simulink model "Exp13_CCCV"  (R2022b)
settings: Solver=VariableStepAuto  StartTime=0.0  StopTime=3600  RelTol=1e-3
undefined symbols (not defined in the file or in its folder): Ion, Lithium
libraries: spsBatteryLib x3, BatteryCurrentManagement x2, spsControlledCurrentSourceLib x2, spsDiodeLib x2, spsIdealSwitchLib x2, spsSeriesRLCBranchLib x2, spsGroundLib x1, BatteryBalancing x1, sps_lib x1
settings Model: Creator=SASTRA  LastModifiedBy=SASTRA
settings SolverCC: MaxConsecutiveMinStep=100

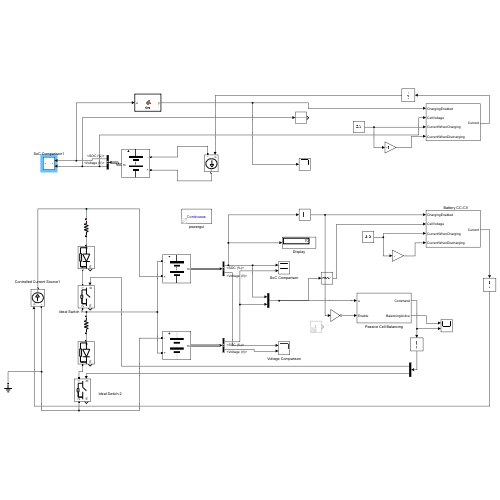
[thumbnail: Simulink's stored preview of the top-level diagram]
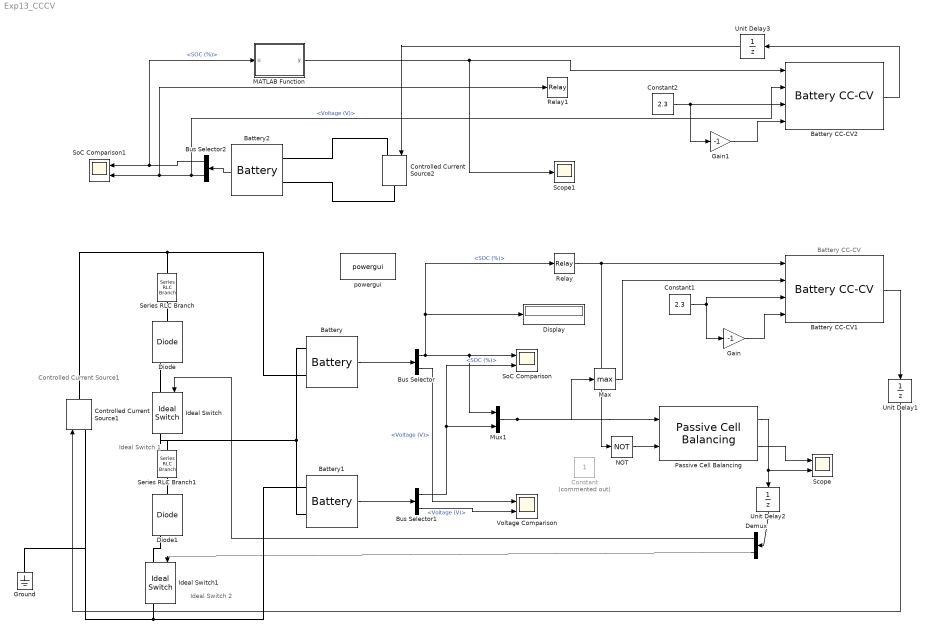
== system Exp13_CCCV ==
  note: Ideal Switch 1
  note: Ideal Switch 2
  note: Controlled Current Source1
  note: Battery CC-CV
  Battery : spsBatteryLib/Battery  BatType=Lithium-Ion  ShowTempParam=off  ThermalPreset="3.3V  2.3Ah  (LiFePO4)"  ShowAgeParam=off  NomV=3.1  NomQ=2.3  SOC=70  Batt_Tr=1  PresetModel=off  MaxQ=2.3  MinV=3.75  FullV=3.748  Dis_rate=2.3  R=0.014  Normal_OP=2.25  expZone="[3.4788       0.113]"  current=[6.5 13 32.5]  Units=Time  Tci=20  NomT=25  T2=0  MaxQ2=2.208  FullV2=3.45  Normal_OP2=2.85  expZone2="[3.22       0.015]"  Rca=0.6  ti=1000  Dp=0  Neq0=0  Tsim=1e6  Ta1=25  Qeol=5.4*0.9  Reol=0.013333*1.2  Char_age=[2.3478, 3]  Dis_age=[2.3478, 10]  N1=1500  N2=10500  N3=1000  N4=1400  Ta2=45  N5=950
  Battery CC-CV1 : BatteryCurrentManagement/Battery CC-CV  MaxCellVoltage=4.5  Kp=100  Ki=10  Kaw=1  Ts=1
      settings: LibrarySourceBlock=batt_sl_lib/Current Management/Battery CC-CV
  Battery CC-CV2 : BatteryCurrentManagement/Battery CC-CV  MaxCellVoltage=4.5  Kp=100  Ki=10  Kaw=1  Ts=1
      settings: LibrarySourceBlock=batt_sl_lib/Current Management/Battery CC-CV
  Battery1 : spsBatteryLib/Battery  BatType=Lithium-Ion  ShowTempParam=off  ThermalPreset="3.3V  2.3Ah  (LiFePO4)"  ShowAgeParam=off  NomV=3.1  NomQ=2.3  SOC=50  Batt_Tr=1  PresetModel=off  MaxQ=2.3  MinV=2.475  FullV=3.748  Dis_rate=2.3  R=0.014  Normal_OP=2.25  expZone="[3.4788       0.113]"  current=[6.5 13 32.5]  Units=Time  Tci=20  NomT=25  T2=0  MaxQ2=2.208  FullV2=3.45  Normal_OP2=2.85  expZone2="[3.22       0.015]"  Rca=0.6  ti=1000  Dp=0  Neq0=0  Tsim=1e6  Ta1=25  Qeol=5.4*0.9  Reol=0.013333*1.2  Char_age=[2.3478, 3]  Dis_age=[2.3478, 10]  N1=1500  N2=10500  N3=1000  N4=1400  Ta2=45  N5=950
  Battery2 : spsBatteryLib/Battery  BatType=Lithium-Ion  ShowTempParam=off  ThermalPreset="3.3V  2.3Ah  (LiFePO4)"  ShowAgeParam=off  NomV=3.1  NomQ=2.3  SOC=70  Batt_Tr=1  PresetModel=off  MaxQ=2.3  MinV=3.75  FullV=3.748  Dis_rate=2.3  R=0.014  Normal_OP=2.25  expZone="[3.4788       0.113]"  current=[6.5 13 32.5]  Units=Time  Tci=20  NomT=25  T2=0  MaxQ2=2.208  FullV2=3.45  Normal_OP2=2.85  expZone2="[3.22       0.015]"  Rca=0.6  ti=1000  Dp=0  Neq0=0  Tsim=1e6  Ta1=25  Qeol=5.4*0.9  Reol=0.013333*1.2  Char_age=[2.3478, 3]  Dis_age=[2.3478, 10]  N1=1500  N2=10500  N3=1000  N4=1400  Ta2=45  N5=950
  Bus Selector : BusSelector  OutputSignals=SOC (%),Voltage (V)
  Bus Selector1 : BusSelector  OutputSignals=SOC (%),Voltage (V)
  Bus Selector2 : BusSelector  OutputSignals=SOC (%),Voltage (V)
  Constant : Constant  Commented=on
  Constant1 : Constant  Value=2.3
  Constant2 : Constant  Value=2.3
  Controlled Current Source1 : spsControlledCurrentSourceLib/Controlled Current Source  Initialize=on  Source_Type=DC  Amplitude=0  Phase=0  Frequency=0  Measurements=Current
  Controlled Current Source2 : spsControlledCurrentSourceLib/Controlled Current Source  Initialize=on  Source_Type=DC  Amplitude=0  Phase=0  Frequency=0  Measurements=Current
  Demux : Demux  Outputs=2
  Diode : spsDiodeLib/Diode  Ron=0.001  Lon=0  Vf=0.8  IC=0  UseSnubber=0  Rs=500  Cs=250e-9  Measurements=on
  Diode1 : spsDiodeLib/Diode  Ron=0.001  Lon=0  Vf=0.8  IC=0  UseSnubber=0  Rs=500  Cs=250e-9  Measurements=on
  Display : Display
  Gain : Gain  Gain=-1
  Gain1 : Gain  Gain=-1
  Ground : spsGroundLib/Ground  LConnTagsString=a
  Ideal Switch : spsIdealSwitchLib/Ideal Switch  Ron=0.001  Lon=0  IC=0  Rs=1e5  Cs=inf  Measurements=on
  Ideal Switch1 : spsIdealSwitchLib/Ideal Switch  Ron=0.001  Lon=0  IC=0  Rs=1e5  Cs=inf  Measurements=on
  MATLAB Function : MATLAB Function  TreatAsAtomicUnit=on
  Max : MinMax  Function=max
  Mux1 : Mux  Inputs=2
  NOT : Logic  Operator=NOT  IconShape=distinctive  AllPortsSameDT=off  OutDataTypeStr=boolean
  Passive Cell Balancing : BatteryBalancing/Passive Cell Balancing  Threshold=0.2  Td_on=1  Td_off=1  Ts=1
      settings: LibrarySourceBlock=batt_sl_lib/Cell Balancing/Passive Cell Balancing
  Relay : Relay  OnSwitchValue=90  OffSwitchValue=30  OnOutputValue=0  OffOutputValue=1
  Relay1 : Relay  OnSwitchValue=3.3  OffSwitchValue=3.2
  Scope : Scope  NumInputPorts=2
  Scope1 : Scope
  Series RLC Branch : spsSeriesRLCBranchLib/Series RLC Branch  LConnTagsString=__new0  RConnTagsString=__new0  BranchType=R  Resistance=10  Inductance=1e-3  SetiL0=off  InitialCurrent=0  Capacitance=1e-6  Setx0=off  InitialVoltage=0  Measurements=None
  Series RLC Branch1 : spsSeriesRLCBranchLib/Series RLC Branch  LConnTagsString=__new0  RConnTagsString=__new0  BranchType=R  Resistance=10  Inductance=1e-3  SetiL0=off  InitialCurrent=0  Capacitance=1e-6  Setx0=off  InitialVoltage=0  Measurements=None
  SoC Comparison : Scope  NumInputPorts=2
  SoC Comparison1 : Scope  NumInputPorts=2
  Unit Delay1 : UnitDelay  SampleTime=-1  HasFrameUpgradeWarning=on
  Unit Delay2 : UnitDelay  SampleTime=-1  HasFrameUpgradeWarning=on
  Unit Delay3 : UnitDelay  SampleTime=-1  HasFrameUpgradeWarning=on
  Voltage Comparison : Scope  NumInputPorts=2
  powergui : sps_lib/powergui  Priority=1  SimulationMode=Continuous  SampleTime=50e-6  frequency=60  Iterations=50  frequencyindice=0  Pbase=100e6  ErrMax=1e-4  UnitsV=kV  UnitsW=MW  buscounter=0  FunctionMessages=off  echomessages=off  EnableUseOfTLC=off  CurrentSourceSwitches=off  DisableSnubberDevices=off  DisableRonSwitches=off  DisableVfSwitches=off  DisplayEquations=off  AutomaticDiscreteSolvers=off  SolverType=Tustin/Backward Euler (TBE)  Interpol=off  ExternalGateDelay=off  methode=off  Ts=100  x0status=blocks  SPID=on  SwTol=0  HookPort=off  NonlinearTolerance=1e-4  nMaxIteration=100  ContinueOnMaxIteration=off  RestoreLinks=warning  ResistiveCurrentMeasurement=off  Frange=[0:2:500]  Ylog=off  Xlog=on  ShowGrid=off  save=off  variable=ZData  structure=0  ZoomFFT=off  StartTime=0.0  cycles=1  DisplayStyle=1  fundamental=60  FreqAxis=off  MaxFrequency=1000  frequencyindicesteady=1  RmsSteady=1  display=off
  wires:
  Battery/1 -> Bus Selector/1
  Battery1/1 -> Bus Selector1/1
  Bus Selector/1 -> Display/1, Relay/1, Mux1/1, SoC Comparison/1  "<SOC (%)>"
  Bus Selector1/1 -> Mux1/2, SoC Comparison/2  "<SOC (%)>"
  Passive Cell Balancing/1 -> Unit Delay2/1, Scope/2
  Demux/1 -> Ideal Switch/1
  Demux/2 -> Ideal Switch1/1
  Passive Cell Balancing/2 -> Scope/1
  Relay/1 -> NOT/1, Battery CC-CV1/1
  Mux1/1 -> Passive Cell Balancing/1, Max/1
  Max/1 -> Battery CC-CV1/2
  Constant1/1 -> Gain/1, Battery CC-CV1/3
  Gain/1 -> Battery CC-CV1/4
  Battery CC-CV1/1 -> Unit Delay1/1
  Unit Delay2/1 -> Demux/1
  Unit Delay1/1 -> Controlled Current Source1/1
  Bus Selector/2 -> Voltage Comparison/1  "<Voltage (V)>"
  Bus Selector1/2 -> Voltage Comparison/2  "<Voltage (V)>"
  NOT/1 -> Passive Cell Balancing/2
  Battery2/1 -> Bus Selector2/1
  Constant2/1 -> Gain1/1, Battery CC-CV2/3
  Gain1/1 -> Battery CC-CV2/4
  Battery CC-CV2/1 -> Unit Delay3/1
  Bus Selector2/1 -> MATLAB Function/1(u), SoC Comparison1/1  "<SOC (%)>"
  MATLAB Function/1(y) -> Scope1/1, Battery CC-CV2/1
  Bus Selector2/2 -> Battery CC-CV2/2, Relay1/1, SoC Comparison1/2  "<Voltage (V)>"
  Unit Delay3/1 -> Controlled Current Source2/1
  connections:
  Battery/LConn2 -- Series RLC Branch1/LConn1 -- Ideal Switch/RConn1 -- Battery1/LConn1
  Series RLC Branch/LConn1 -- Controlled Current Source1/RConn1 -- Battery/LConn1
  Ideal Switch1/RConn1 -- Controlled Current Source1/LConn1 -- Ground/LConn1 -- Battery1/LConn2
  Diode/RConn1 -- Ideal Switch/LConn1
  Diode1/RConn1 -- Ideal Switch1/LConn1
  Series RLC Branch/RConn1 -- Diode/LConn1
  Diode1/LConn1 -- Series RLC Branch1/RConn1
  Battery2/LConn1 -- Controlled Current Source2/RConn1
  Battery2/LConn2 -- Controlled Current Source2/LConn1

== matlab function Exp13_CCCV/MATLAB Function ==
  data: u input; y output
function y = fcn(u)
if(u>95)
    y=0;
else 
    y=1;
end 
end
